simulink model "SWC_CGW_type"  (R2021b)
settings: Solver=FixedStepDiscrete  StartTime=0.0  StopTime=10.0  RelTol=1e-3
(part 2 of 3)

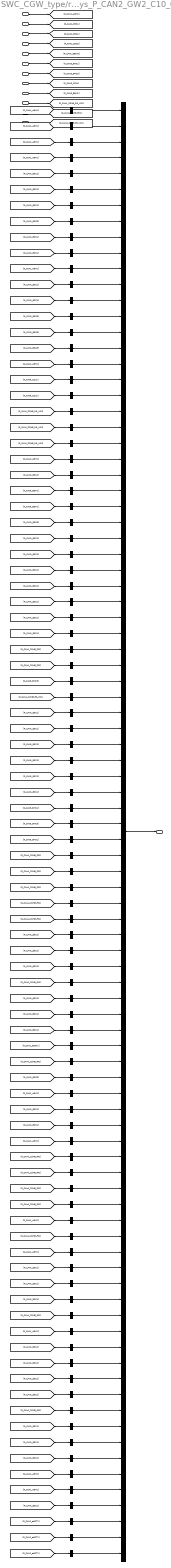
== system SWC_CGW_type/run_SWC_CGW_sys/CGW/Sys_P_CAN2_GW2_C10_0 ==
  R_CAN1_ABM1 : Inport
  R_CAN1_EPS1 : Inport  Port=2
  R_CAN1_ESC1 : Inport  Port=3
  R_CAN1_ESC5 : Inport  Port=4
  R_CAN1_eBST1 : Inport  Port=5
  R_CAN3_BMS1 : Inport  Port=6
  R_CAN3_BMS3 : Inport  Port=7
  R_CAN3_CCU1 : Inport  Port=8
  R_CAN3_EBM1 : Inport  Port=9
  R_CAN4_ZONE_DR_VCU : Inport  Port=10
  R_CAN4_ZONE_FR1 : Inport  Port=11
  R_CAN4_ZONE_FR_VCU : Inport  Port=12
  bus_creator : BusCreator  Inputs=92  OutDataTypeStr=Bus: DT_CAN2_SG_GW2_C10_0  NonVirtualBus=on
  bus_selector : BusSelector  OutputSignals=CAN1_ABM_Passenger_ODS_Sta
  bus_selector1 : BusSelector  OutputSignals=CAN1_ABM_RearPassengerCTR_ODS_Sta
  bus_selector10 : BusSelector  OutputSignals=CAN1_AirBagFailCmd
  bus_selector11 : BusSelector  OutputSignals=CAN1_Amber_WnlmpSta
  bus_selector12 : BusSelector  OutputSignals=CAN1_BTCS_Active
  bus_selector13 : BusSelector  OutputSignals=CAN1_BrkDiscTempSta
  bus_selector14 : BusSelector  OutputSignals=CAN1_BrkSw_Sta
  bus_selector15 : BusSelector  OutputSignals=CAN1_BrkSw_V
  bus_selector16 : BusSelector  OutputSignals=CAN1_CrashOutputSts
  bus_selector17 : BusSelector  OutputSignals=CAN3_DCDCAuxCur
  bus_selector18 : BusSelector  OutputSignals=CAN3_DCDCAuxVolt
  bus_selector19 : BusSelector  OutputSignals=CAN4_DrPMMLVOutPErrLmp
  bus_selector2 : BusSelector  OutputSignals=CAN1_ABM_RearPassengerLH_ODS_Sta
  bus_selector20 : BusSelector  OutputSignals=CAN4_DrPMMSysErrLmp
  bus_selector21 : BusSelector  OutputSignals=CAN4_DrSCPSysErrLmp
  bus_selector22 : BusSelector  OutputSignals=CAN1_DriverSeatBeltCmd
  bus_selector23 : BusSelector  OutputSignals=CAN1_EBD_Failed
  bus_selector24 : BusSelector  OutputSignals=CAN3_EBMErrSta
  bus_selector25 : BusSelector  OutputSignals=CAN3_EBMRLampSta
  bus_selector26 : BusSelector  OutputSignals=CAN1_ESC_ADAS_Sta
  bus_selector27 : BusSelector  OutputSignals=CAN1_ESC_BeepReq
  bus_selector28 : BusSelector  OutputSignals=CAN1_ESC_Failed
  bus_selector29 : BusSelector  OutputSignals=CAN1_ESC_OFF_Status
  bus_selector3 : BusSelector  OutputSignals=CAN1_ABM_RearPassengerRH_ODS_Sta
  bus_selector30 : BusSelector  OutputSignals=CAN1_ESC_Off_lmpSta
  bus_selector31 : BusSelector  OutputSignals=CAN1_ESC_WnlmpSta
  bus_selector32 : BusSelector  OutputSignals=CAN1_ESS_Active
  bus_selector33 : BusSelector  OutputSignals=CAN1_EpasFailed
  bus_selector34 : BusSelector  OutputSignals=CAN4_FLTurn_Light_Warning
  bus_selector35 : BusSelector  OutputSignals=CAN4_FRTurn_Light_Warning
  bus_selector36 : BusSelector  OutputSignals=CAN3_FireDetErr
  bus_selector37 : BusSelector  OutputSignals=CAN4_FrPMMLimpHomeActReq
  bus_selector38 : BusSelector  OutputSignals=CAN1_HBB_Active
  bus_selector39 : BusSelector  OutputSignals=CAN1_HBB_Failed
  bus_selector4 : BusSelector  OutputSignals=CAN1_ABS_Active
  bus_selector40 : BusSelector  OutputSignals=CAN1_HDD_Active
  bus_selector41 : BusSelector  OutputSignals=CAN1_HDD_Failed
  bus_selector42 : BusSelector  OutputSignals=CAN1_HSA_Active
  bus_selector43 : BusSelector  OutputSignals=CAN1_HSA_Failed
  bus_selector44 : BusSelector  OutputSignals=CAN3_HVBattCurr
  bus_selector45 : BusSelector  OutputSignals=CAN3_HVBattErr
  bus_selector46 : BusSelector  OutputSignals=CAN3_HVBattVolt
  bus_selector47 : BusSelector  OutputSignals=CAN4_LADB_Hibeam_Indication
  bus_selector48 : BusSelector  OutputSignals=CAN4_LADB_Operation_Status
  bus_selector49 : BusSelector  OutputSignals=CAN4_LADB_Warning
  bus_selector5 : BusSelector  OutputSignals=CAN1_ABS_Failed
  bus_selector50 : BusSelector  OutputSignals=CAN4_LAHB_Warning
  bus_selector51 : BusSelector  OutputSignals=CAN4_LDRL_Warning
  bus_selector52 : BusSelector  OutputSignals=CAN1_LF_PulseCount
  bus_selector53 : BusSelector  OutputSignals=CAN1_LF_PulseCount_V
  bus_selector54 : BusSelector  OutputSignals=CAN1_LF_WhlRotDir
  bus_selector55 : BusSelector  OutputSignals=CAN4_LLB_Warning
  bus_selector56 : BusSelector  OutputSignals=CAN1_LR_PulseCount
  bus_selector57 : BusSelector  OutputSignals=CAN1_LR_PulseCount_V
  bus_selector58 : BusSelector  OutputSignals=CAN1_LR_WhlRotDir
  bus_selector59 : BusSelector  OutputSignals=CAN1_LowBrakeFluid_Sta
  bus_selector6 : BusSelector  OutputSignals=CAN1_ABS_WnlmpSta
  bus_selector60 : BusSelector  OutputSignals=CAN4_Lposition_Lamp_Warning
  bus_selector61 : BusSelector  OutputSignals=CAN1_Meter_Ind_VehSpeed
  bus_selector62 : BusSelector  OutputSignals=CAN1_PABSwitchCmd
  bus_selector63 : BusSelector  OutputSignals=CAN1_PBA_Active
  bus_selector64 : BusSelector  OutputSignals=CAN1_PBA_Failed
  bus_selector65 : BusSelector  OutputSignals=CAN1_PsngrSeatBeltCmd
  bus_selector66 : BusSelector  OutputSignals=CAN4_RADB_Hibeam_Indication
  bus_selector67 : BusSelector  OutputSignals=CAN4_RADB_Operation_Status
  bus_selector68 : BusSelector  OutputSignals=CAN4_RADB_Warning
  bus_selector69 : BusSelector  OutputSignals=CAN4_RAHB_Warning
  bus_selector7 : BusSelector  OutputSignals=CAN1_AEBAvail
  bus_selector70 : BusSelector  OutputSignals=CAN1_RCenterSeatBeltCmd
  bus_selector71 : BusSelector  OutputSignals=CAN4_RDRL_Warning
  bus_selector72 : BusSelector  OutputSignals=CAN1_RDriverSeatBeltCmd
  bus_selector73 : BusSelector  OutputSignals=CAN1_RF_PulseCount
  bus_selector74 : BusSelector  OutputSignals=CAN1_RF_PulseCount_V
  bus_selector75 : BusSelector  OutputSignals=CAN1_RF_WhlRotDir
  bus_selector76 : BusSelector  OutputSignals=CAN4_RLB_Warning
  bus_selector77 : BusSelector  OutputSignals=CAN1_RPsngrSeatBeltCmd
  bus_selector78 : BusSelector  OutputSignals=CAN1_RR_PulseCount
  bus_selector79 : BusSelector  OutputSignals=CAN1_RR_PulseCount_V
  bus_selector8 : BusSelector  OutputSignals=CAN1_AVH_Active
  bus_selector80 : BusSelector  OutputSignals=CAN1_RR_WhlRotDir
  bus_selector81 : BusSelector  OutputSignals=CAN1_Red_WnlmpSta
  bus_selector82 : BusSelector  OutputSignals=CAN4_Rposition_Lamp_Warning
  bus_selector83 : BusSelector  OutputSignals=CAN1_SAS_Angle
  bus_selector84 : BusSelector  OutputSignals=CAN1_SAS_V
  bus_selector85 : BusSelector  OutputSignals=CAN1_TCS_Failed
  bus_selector86 : BusSelector  OutputSignals=CAN1_TLHPsngrSeatBeltCmd
  bus_selector87 : BusSelector  OutputSignals=CAN1_TRHPsngrSeatBeltCmd
  bus_selector88 : BusSelector  OutputSignals=CAN1_VehSpeed
  bus_selector89 : BusSelector  OutputSignals=CAN1_eBST_AmberWnlmpSta
  bus_selector9 : BusSelector  OutputSignals=CAN1_AVH_Failed
  bus_selector90 : BusSelector  OutputSignals=CAN1_eBST_BeepReq
  bus_selector91 : BusSelector  OutputSignals=CAN1_eBST_RedWnlmpSta
  P_CAN2_GW2_C10_0 : Outport
  wires:
  bus_creator/1 -> P_CAN2_GW2_C10_0/1
  bus_selector/1 -> bus_creator/1  "<CAN1_ABM_Passenger_ODS_Sta>"
  [R_CAN1_ABM1] -> bus_selector/1
  bus_selector1/1 -> bus_creator/2  "<CAN1_ABM_RearPassengerCTR_ODS_Sta>"
  [R_CAN1_ABM1] -> bus_selector1/1
  bus_selector2/1 -> bus_creator/3  "<CAN1_ABM_RearPassengerLH_ODS_Sta>"
  [R_CAN1_ABM1] -> bus_selector2/1
  bus_selector3/1 -> bus_creator/4  "<CAN1_ABM_RearPassengerRH_ODS_Sta>"
  [R_CAN1_ABM1] -> bus_selector3/1
  bus_selector4/1 -> bus_creator/5  "<CAN1_ABS_Active>"
  [R_CAN1_ESC1] -> bus_selector4/1
  bus_selector5/1 -> bus_creator/6  "<CAN1_ABS_Failed>"
  [R_CAN1_ESC1] -> bus_selector5/1
  bus_selector6/1 -> bus_creator/7  "<CAN1_ABS_WnlmpSta>"
  [R_CAN1_ESC1] -> bus_selector6/1
  bus_selector7/1 -> bus_creator/8  "<CAN1_AEBAvail>"
  [R_CAN1_ESC5] -> bus_selector7/1
  bus_selector8/1 -> bus_creator/9  "<CAN1_AVH_Active>"
  [R_CAN1_ESC1] -> bus_selector8/1
  bus_selector9/1 -> bus_creator/10  "<CAN1_AVH_Failed>"
  [R_CAN1_ESC1] -> bus_selector9/1
  bus_selector10/1 -> bus_creator/11  "<CAN1_AirBagFailCmd>"
  [R_CAN1_ABM1] -> bus_selector10/1
  bus_selector11/1 -> bus_creator/12  "<CAN1_Amber_WnlmpSta>"
  [R_CAN1_ESC1] -> bus_selector11/1
  bus_selector12/1 -> bus_creator/13  "<CAN1_BTCS_Active>"
  [R_CAN1_ESC1] -> bus_selector12/1
  bus_selector13/1 -> bus_creator/14  "<CAN1_BrkDiscTempSta>"
  [R_CAN1_ESC5] -> bus_selector13/1
  bus_selector14/1 -> bus_creator/15  "<CAN1_BrkSw_Sta>"
  [R_CAN1_ESC5] -> bus_selector14/1
  bus_selector15/1 -> bus_creator/16  "<CAN1_BrkSw_V>"
  [R_CAN1_ESC5] -> bus_selector15/1
  bus_selector16/1 -> bus_creator/17  "<CAN1_CrashOutputSts>"
  [R_CAN1_ABM1] -> bus_selector16/1
  bus_selector17/1 -> bus_creator/18  "<CAN3_DCDCAuxCur>"
  [R_CAN3_CCU1] -> bus_selector17/1
  bus_selector18/1 -> bus_creator/19  "<CAN3_DCDCAuxVolt>"
  [R_CAN3_CCU1] -> bus_selector18/1
  bus_selector19/1 -> bus_creator/20  "<CAN4_DrPMMLVOutPErrLmp>"
  [R_CAN4_ZONE_DR_VCU] -> bus_selector19/1
  bus_selector20/1 -> bus_creator/21  "<CAN4_DrPMMSysErrLmp>"
  [R_CAN4_ZONE_DR_VCU] -> bus_selector20/1
  bus_selector21/1 -> bus_creator/22  "<CAN4_DrSCPSysErrLmp>"
  [R_CAN4_ZONE_DR_VCU] -> bus_selector21/1
  bus_selector22/1 -> bus_creator/23  "<CAN1_DriverSeatBeltCmd>"
  [R_CAN1_ABM1] -> bus_selector22/1
  bus_selector23/1 -> bus_creator/24  "<CAN1_EBD_Failed>"
  [R_CAN1_ESC1] -> bus_selector23/1
  bus_selector24/1 -> bus_creator/25  "<CAN3_EBMErrSta>"
  [R_CAN3_EBM1] -> bus_selector24/1
  bus_selector25/1 -> bus_creator/26  "<CAN3_EBMRLampSta>"
  [R_CAN3_EBM1] -> bus_selector25/1
  bus_selector26/1 -> bus_creator/27  "<CAN1_ESC_ADAS_Sta>"
  [R_CAN1_ESC5] -> bus_selector26/1
  bus_selector27/1 -> bus_creator/28  "<CAN1_ESC_BeepReq>"
  [R_CAN1_ESC1] -> bus_selector27/1
  bus_selector28/1 -> bus_creator/29  "<CAN1_ESC_Failed>"
  [R_CAN1_ESC1] -> bus_selector28/1
  bus_selector29/1 -> bus_creator/30  "<CAN1_ESC_OFF_Status>"
  [R_CAN1_ESC1] -> bus_selector29/1
  bus_selector30/1 -> bus_creator/31  "<CAN1_ESC_Off_lmpSta>"
  [R_CAN1_ESC1] -> bus_selector30/1
  bus_selector31/1 -> bus_creator/32  "<CAN1_ESC_WnlmpSta>"
  [R_CAN1_ESC1] -> bus_selector31/1
  bus_selector32/1 -> bus_creator/33  "<CAN1_ESS_Active>"
  [R_CAN1_ESC1] -> bus_selector32/1
  bus_selector33/1 -> bus_creator/34  "<CAN1_EpasFailed>"
  [R_CAN1_EPS1] -> bus_selector33/1
  bus_selector34/1 -> bus_creator/35  "<CAN4_FLTurn_Light_Warning>"
  [R_CAN4_ZONE_FR1] -> bus_selector34/1
  bus_selector35/1 -> bus_creator/36  "<CAN4_FRTurn_Light_Warning>"
  [R_CAN4_ZONE_FR1] -> bus_selector35/1
  bus_selector36/1 -> bus_creator/37  "<CAN3_FireDetErr>"
  [R_CAN3_BMS3] -> bus_selector36/1
  bus_selector37/1 -> bus_creator/38  "<CAN4_FrPMMLimpHomeActReq>"
  [R_CAN4_ZONE_FR_VCU] -> bus_selector37/1
  bus_selector38/1 -> bus_creator/39  "<CAN1_HBB_Active>"
  [R_CAN1_ESC1] -> bus_selector38/1
  bus_selector39/1 -> bus_creator/40  "<CAN1_HBB_Failed>"
  [R_CAN1_ESC1] -> bus_selector39/1
  bus_selector40/1 -> bus_creator/41  "<CAN1_HDD_Active>"
  [R_CAN1_ESC1] -> bus_selector40/1
  bus_selector41/1 -> bus_creator/42  "<CAN1_HDD_Failed>"
  [R_CAN1_ESC1] -> bus_selector41/1
  bus_selector42/1 -> bus_creator/43  "<CAN1_HSA_Active>"
  [R_CAN1_ESC1] -> bus_selector42/1
  bus_selector43/1 -> bus_creator/44  "<CAN1_HSA_Failed>"
  [R_CAN1_ESC1] -> bus_selector43/1
  bus_selector44/1 -> bus_creator/45  "<CAN3_HVBattCurr>"
  [R_CAN3_BMS1] -> bus_selector44/1
  bus_selector45/1 -> bus_creator/46  "<CAN3_HVBattErr>"
  [R_CAN3_BMS3] -> bus_selector45/1
  bus_selector46/1 -> bus_creator/47  "<CAN3_HVBattVolt>"
  [R_CAN3_BMS1] -> bus_selector46/1
  bus_selector47/1 -> bus_creator/48  "<CAN4_LADB_Hibeam_Indication>"
  [R_CAN4_ZONE_FR1] -> bus_selector47/1
  bus_selector48/1 -> bus_creator/49  "<CAN4_LADB_Operation_Status>"
  [R_CAN4_ZONE_FR1] -> bus_selector48/1
  bus_selector49/1 -> bus_creator/50  "<CAN4_LADB_Warning>"
  [R_CAN4_ZONE_FR1] -> bus_selector49/1
  bus_selector50/1 -> bus_creator/51  "<CAN4_LAHB_Warning>"
  [R_CAN4_ZONE_FR1] -> bus_selector50/1
  bus_selector51/1 -> bus_creator/52  "<CAN4_LDRL_Warning>"
  [R_CAN4_ZONE_FR1] -> bus_selector51/1
  bus_selector52/1 -> bus_creator/53  "<CAN1_LF_PulseCount>"
  [R_CAN1_ESC1] -> bus_selector52/1
  bus_selector53/1 -> bus_creator/54  "<CAN1_LF_PulseCount_V>"
  [R_CAN1_ESC1] -> bus_selector53/1
  bus_selector54/1 -> bus_creator/55  "<CAN1_LF_WhlRotDir>"
  [R_CAN1_ESC1] -> bus_selector54/1
  bus_selector55/1 -> bus_creator/56  "<CAN4_LLB_Warning>"
  [R_CAN4_ZONE_FR1] -> bus_selector55/1
  bus_selector56/1 -> bus_creator/57  "<CAN1_LR_PulseCount>"
  [R_CAN1_ESC1] -> bus_selector56/1
  bus_selector57/1 -> bus_creator/58  "<CAN1_LR_PulseCount_V>"
  [R_CAN1_ESC1] -> bus_selector57/1
  bus_selector58/1 -> bus_creator/59  "<CAN1_LR_WhlRotDir>"
  [R_CAN1_ESC1] -> bus_selector58/1
  bus_selector59/1 -> bus_creator/60  "<CAN1_LowBrakeFluid_Sta>"
  [R_CAN1_eBST1] -> bus_selector59/1
  bus_selector60/1 -> bus_creator/61  "<CAN4_Lposition_Lamp_Warning>"
  [R_CAN4_ZONE_FR1] -> bus_selector60/1
  bus_selector61/1 -> bus_creator/62  "<CAN1_Meter_Ind_VehSpeed>"
  [R_CAN1_ESC5] -> bus_selector61/1
  bus_selector62/1 -> bus_creator/63  "<CAN1_PABSwitchCmd>"
  [R_CAN1_ABM1] -> bus_selector62/1
  bus_selector63/1 -> bus_creator/64  "<CAN1_PBA_Active>"
  [R_CAN1_ESC1] -> bus_selector63/1
  bus_selector64/1 -> bus_creator/65  "<CAN1_PBA_Failed>"
  [R_CAN1_ESC1] -> bus_selector64/1
  bus_selector65/1 -> bus_creator/66  "<CAN1_PsngrSeatBeltCmd>"
  [R_CAN1_ABM1] -> bus_selector65/1
  bus_selector66/1 -> bus_creator/67  "<CAN4_RADB_Hibeam_Indication>"
  [R_CAN4_ZONE_FR1] -> bus_selector66/1
  bus_selector67/1 -> bus_creator/68  "<CAN4_RADB_Operation_Status>"
  [R_CAN4_ZONE_FR1] -> bus_selector67/1
  bus_selector68/1 -> bus_creator/69  "<CAN4_RADB_Warning>"
  [R_CAN4_ZONE_FR1] -> bus_selector68/1
  bus_selector69/1 -> bus_creator/70  "<CAN4_RAHB_Warning>"
  [R_CAN4_ZONE_FR1] -> bus_selector69/1
  bus_selector70/1 -> bus_creator/71  "<CAN1_RCenterSeatBeltCmd>"
  [R_CAN1_ABM1] -> bus_selector70/1
  bus_selector71/1 -> bus_creator/72  "<CAN4_RDRL_Warning>"
  [R_CAN4_ZONE_FR1] -> bus_selector71/1
  bus_selector72/1 -> bus_creator/73  "<CAN1_RDriverSeatBeltCmd>"
  [R_CAN1_ABM1] -> bus_selector72/1
  bus_selector73/1 -> bus_creator/74  "<CAN1_RF_PulseCount>"
  [R_CAN1_ESC1] -> bus_selector73/1
  bus_selector74/1 -> bus_creator/75  "<CAN1_RF_PulseCount_V>"
  [R_CAN1_ESC1] -> bus_selector74/1
  bus_selector75/1 -> bus_creator/76  "<CAN1_RF_WhlRotDir>"
  [R_CAN1_ESC1] -> bus_selector75/1
  bus_selector76/1 -> bus_creator/77  "<CAN4_RLB_Warning>"
  [R_CAN4_ZONE_FR1] -> bus_selector76/1
  bus_selector77/1 -> bus_creator/78  "<CAN1_RPsngrSeatBeltCmd>"
  [R_CAN1_ABM1] -> bus_selector77/1
  bus_selector78/1 -> bus_creator/79  "<CAN1_RR_PulseCount>"
  [R_CAN1_ESC1] -> bus_selector78/1
  bus_selector79/1 -> bus_creator/80  "<CAN1_RR_PulseCount_V>"
  [R_CAN1_ESC1] -> bus_selector79/1
  bus_selector80/1 -> bus_creator/81  "<CAN1_RR_WhlRotDir>"
  [R_CAN1_ESC1] -> bus_selector80/1
  bus_selector81/1 -> bus_creator/82  "<CAN1_Red_WnlmpSta>"
  [R_CAN1_ESC1] -> bus_selector81/1
  bus_selector82/1 -> bus_creator/83  "<CAN4_Rposition_Lamp_Warning>"
  [R_CAN4_ZONE_FR1] -> bus_selector82/1
  bus_selector83/1 -> bus_creator/84  "<CAN1_SAS_Angle>"
  [R_CAN1_EPS1] -> bus_selector83/1
  bus_selector84/1 -> bus_creator/85  "<CAN1_SAS_V>"
  [R_CAN1_EPS1] -> bus_selector84/1
  bus_selector85/1 -> bus_creator/86  "<CAN1_TCS_Failed>"
  [R_CAN1_ESC1] -> bus_selector85/1
  bus_selector86/1 -> bus_creator/87  "<CAN1_TLHPsngrSeatBeltCmd>"
  [R_CAN1_ABM1] -> bus_selector86/1
  bus_selector87/1 -> bus_creator/88  "<CAN1_TRHPsngrSeatBeltCmd>"
  [R_CAN1_ABM1] -> bus_selector87/1
  bus_selector88/1 -> bus_creator/89  "<CAN1_VehSpeed>"
  [R_CAN1_ESC1] -> bus_selector88/1
  bus_selector89/1 -> bus_creator/90  "<CAN1_eBST_AmberWnlmpSta>"
  [R_CAN1_eBST1] -> bus_selector89/1
  bus_selector90/1 -> bus_creator/91  "<CAN1_eBST_BeepReq>"
  [R_CAN1_eBST1] -> bus_selector90/1
  bus_selector91/1 -> bus_creator/92  "<CAN1_eBST_RedWnlmpSta>"
  [R_CAN1_eBST1] -> bus_selector91/1
  R_CAN1_ABM1/1 -> [R_CAN1_ABM1]
  R_CAN1_EPS1/1 -> [R_CAN1_EPS1]
  R_CAN1_ESC1/1 -> [R_CAN1_ESC1]
  R_CAN1_ESC5/1 -> [R_CAN1_ESC5]
  R_CAN1_eBST1/1 -> [R_CAN1_eBST1]
  R_CAN3_BMS1/1 -> [R_CAN3_BMS1]
  R_CAN3_BMS3/1 -> [R_CAN3_BMS3]
  R_CAN3_CCU1/1 -> [R_CAN3_CCU1]
  R_CAN3_EBM1/1 -> [R_CAN3_EBM1]
  R_CAN4_ZONE_DR_VCU/1 -> [R_CAN4_ZONE_DR_VCU]
  R_CAN4_ZONE_FR1/1 -> [R_CAN4_ZONE_FR1]
  R_CAN4_ZONE_FR_VCU/1 -> [R_CAN4_ZONE_FR_VCU]

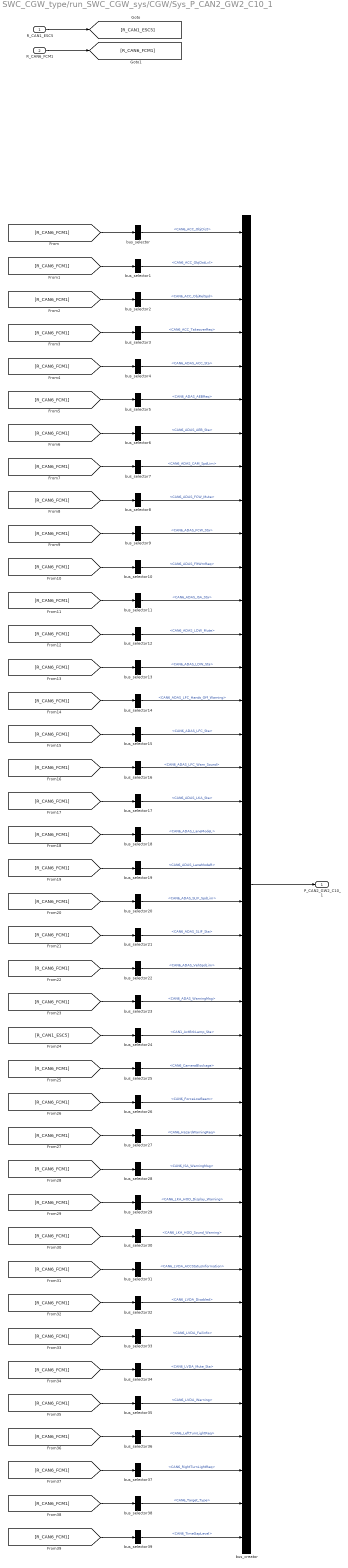
== system SWC_CGW_type/run_SWC_CGW_sys/CGW/Sys_P_CAN2_GW2_C10_1 ==
  R_CAN1_ESC5 : Inport
  R_CAN6_FCM1 : Inport  Port=2
  bus_creator : BusCreator  Inputs=40  OutDataTypeStr=Bus: DT_CAN2_SG_GW2_C10_1  NonVirtualBus=on
  bus_selector : BusSelector  OutputSignals=CAN6_ACC_ObjDist
  bus_selector1 : BusSelector  OutputSignals=CAN6_ACC_ObjDstLvl
  bus_selector10 : BusSelector  OutputSignals=CAN6_ADAS_FltWrnReq
  bus_selector11 : BusSelector  OutputSignals=CAN6_ADAS_ISA_Sta
  bus_selector12 : BusSelector  OutputSignals=CAN6_ADAS_LDW_Mute
  bus_selector13 : BusSelector  OutputSignals=CAN6_ADAS_LDW_Sta
  bus_selector14 : BusSelector  OutputSignals=CAN6_ADAS_LFC_Hands_Off_Warning
  bus_selector15 : BusSelector  OutputSignals=CAN6_ADAS_LFC_Sta
  bus_selector16 : BusSelector  OutputSignals=CAN6_ADAS_LFC_Warn_Sound
  bus_selector17 : BusSelector  OutputSignals=CAN6_ADAS_LKA_Sta
  bus_selector18 : BusSelector  OutputSignals=CAN6_ADAS_LaneModeL
  bus_selector19 : BusSelector  OutputSignals=CAN6_ADAS_LaneModeR
  bus_selector2 : BusSelector  OutputSignals=CAN6_ACC_ObjRelSpd
  bus_selector20 : BusSelector  OutputSignals=CAN6_ADAS_SLIF_SpdLim
  bus_selector21 : BusSelector  OutputSignals=CAN6_ADAS_SLIF_Sta
  bus_selector22 : BusSelector  OutputSignals=CAN6_ADAS_VehSpdLim
  bus_selector23 : BusSelector  OutputSignals=CAN6_ADAS_WarningMsg
  bus_selector24 : BusSelector  OutputSignals=CAN1_ActBrkLamp_Sta
  bus_selector25 : BusSelector  OutputSignals=CAN6_CameraBlockage
  bus_selector26 : BusSelector  OutputSignals=CAN6_ForceLowBeam
  bus_selector27 : BusSelector  OutputSignals=CAN6_HazardWarningReq
  bus_selector28 : BusSelector  OutputSignals=CAN6_ISA_WarningMsg
  bus_selector29 : BusSelector  OutputSignals=CAN6_LKA_HOD_Display_Warning
  bus_selector3 : BusSelector  OutputSignals=CAN6_ACC_TakeoverReq
  bus_selector30 : BusSelector  OutputSignals=CAN6_LKA_HOD_Sound_Warning
  bus_selector31 : BusSelector  OutputSignals=CAN6_LVDA_ACCStatusInformation
  bus_selector32 : BusSelector  OutputSignals=CAN6_LVDA_Disabled
  bus_selector33 : BusSelector  OutputSignals=CAN6_LVDA_Failinfo
  bus_selector34 : BusSelector  OutputSignals=CAN6_LVDA_Mute_Sta
  bus_selector35 : BusSelector  OutputSignals=CAN6_LVDA_Warning
  bus_selector36 : BusSelector  OutputSignals=CAN6_LeftTurnLightReq
  bus_selector37 : BusSelector  OutputSignals=CAN6_RightTurnLightReq
  bus_selector38 : BusSelector  OutputSignals=CAN6_Target_Type
  bus_selector39 : BusSelector  OutputSignals=CAN6_TimeGapLevel
  bus_selector4 : BusSelector  OutputSignals=CAN6_ADAS_ACC_Sta
  bus_selector5 : BusSelector  OutputSignals=CAN6_ADAS_AEBReq
  bus_selector6 : BusSelector  OutputSignals=CAN6_ADAS_AEB_Sta
  bus_selector7 : BusSelector  OutputSignals=CAN6_ADAS_CAM_SpdLim
  bus_selector8 : BusSelector  OutputSignals=CAN6_ADAS_FCW_Mute
  bus_selector9 : BusSelector  OutputSignals=CAN6_ADAS_FCW_Sta
  P_CAN2_GW2_C10_1 : Outport
  wires:
  bus_creator/1 -> P_CAN2_GW2_C10_1/1
  bus_selector/1 -> bus_creator/1  "<CAN6_ACC_ObjDist>"
  [R_CAN6_FCM1] -> bus_selector/1
  bus_selector1/1 -> bus_creator/2  "<CAN6_ACC_ObjDstLvl>"
  [R_CAN6_FCM1] -> bus_selector1/1
  bus_selector2/1 -> bus_creator/3  "<CAN6_ACC_ObjRelSpd>"
  [R_CAN6_FCM1] -> bus_selector2/1
  bus_selector3/1 -> bus_creator/4  "<CAN6_ACC_TakeoverReq>"
  [R_CAN6_FCM1] -> bus_selector3/1
  bus_selector4/1 -> bus_creator/5  "<CAN6_ADAS_ACC_Sta>"
  [R_CAN6_FCM1] -> bus_selector4/1
  bus_selector5/1 -> bus_creator/6  "<CAN6_ADAS_AEBReq>"
  [R_CAN6_FCM1] -> bus_selector5/1
  bus_selector6/1 -> bus_creator/7  "<CAN6_ADAS_AEB_Sta>"
  [R_CAN6_FCM1] -> bus_selector6/1
  bus_selector7/1 -> bus_creator/8  "<CAN6_ADAS_CAM_SpdLim>"
  [R_CAN6_FCM1] -> bus_selector7/1
  bus_selector8/1 -> bus_creator/9  "<CAN6_ADAS_FCW_Mute>"
  [R_CAN6_FCM1] -> bus_selector8/1
  bus_selector9/1 -> bus_creator/10  "<CAN6_ADAS_FCW_Sta>"
  [R_CAN6_FCM1] -> bus_selector9/1
  bus_selector10/1 -> bus_creator/11  "<CAN6_ADAS_FltWrnReq>"
  [R_CAN6_FCM1] -> bus_selector10/1
  bus_selector11/1 -> bus_creator/12  "<CAN6_ADAS_ISA_Sta>"
  [R_CAN6_FCM1] -> bus_selector11/1
  bus_selector12/1 -> bus_creator/13  "<CAN6_ADAS_LDW_Mute>"
  [R_CAN6_FCM1] -> bus_selector12/1
  bus_selector13/1 -> bus_creator/14  "<CAN6_ADAS_LDW_Sta>"
  [R_CAN6_FCM1] -> bus_selector13/1
  bus_selector14/1 -> bus_creator/15  "<CAN6_ADAS_LFC_Hands_Off_Warning>"
  [R_CAN6_FCM1] -> bus_selector14/1
  bus_selector15/1 -> bus_creator/16  "<CAN6_ADAS_LFC_Sta>"
  [R_CAN6_FCM1] -> bus_selector15/1
  bus_selector16/1 -> bus_creator/17  "<CAN6_ADAS_LFC_Warn_Sound>"
  [R_CAN6_FCM1] -> bus_selector16/1
  bus_selector17/1 -> bus_creator/18  "<CAN6_ADAS_LKA_Sta>"
  [R_CAN6_FCM1] -> bus_selector17/1
  bus_selector18/1 -> bus_creator/19  "<CAN6_ADAS_LaneModeL>"
  [R_CAN6_FCM1] -> bus_selector18/1
  bus_selector19/1 -> bus_creator/20  "<CAN6_ADAS_LaneModeR>"
  [R_CAN6_FCM1] -> bus_selector19/1
  bus_selector20/1 -> bus_creator/21  "<CAN6_ADAS_SLIF_SpdLim>"
  [R_CAN6_FCM1] -> bus_selector20/1
  bus_selector21/1 -> bus_creator/22  "<CAN6_ADAS_SLIF_Sta>"
  [R_CAN6_FCM1] -> bus_selector21/1
  bus_selector22/1 -> bus_creator/23  "<CAN6_ADAS_VehSpdLim>"
  [R_CAN6_FCM1] -> bus_selector22/1
  bus_selector23/1 -> bus_creator/24  "<CAN6_ADAS_WarningMsg>"
  [R_CAN6_FCM1] -> bus_selector23/1
  bus_selector24/1 -> bus_creator/25  "<CAN1_ActBrkLamp_Sta>"
  [R_CAN1_ESC5] -> bus_selector24/1
  bus_selector25/1 -> bus_creator/26  "<CAN6_CameraBlockage>"
  [R_CAN6_FCM1] -> bus_selector25/1
  bus_selector26/1 -> bus_creator/27  "<CAN6_ForceLowBeam>"
  [R_CAN6_FCM1] -> bus_selector26/1
  bus_selector27/1 -> bus_creator/28  "<CAN6_HazardWarningReq>"
  [R_CAN6_FCM1] -> bus_selector27/1
  bus_selector28/1 -> bus_creator/29  "<CAN6_ISA_WarningMsg>"
  [R_CAN6_FCM1] -> bus_selector28/1
  bus_selector29/1 -> bus_creator/30  "<CAN6_LKA_HOD_Display_Warning>"
  [R_CAN6_FCM1] -> bus_selector29/1
  bus_selector30/1 -> bus_creator/31  "<CAN6_LKA_HOD_Sound_Warning>"
  [R_CAN6_FCM1] -> bus_selector30/1
  bus_selector31/1 -> bus_creator/32  "<CAN6_LVDA_ACCStatusInformation>"
  [R_CAN6_FCM1] -> bus_selector31/1
  bus_selector32/1 -> bus_creator/33  "<CAN6_LVDA_Disabled>"
  [R_CAN6_FCM1] -> bus_selector32/1
  bus_selector33/1 -> bus_creator/34  "<CAN6_LVDA_Failinfo>"
  [R_CAN6_FCM1] -> bus_selector33/1
  bus_selector34/1 -> bus_creator/35  "<CAN6_LVDA_Mute_Sta>"
  [R_CAN6_FCM1] -> bus_selector34/1
  bus_selector35/1 -> bus_creator/36  "<CAN6_LVDA_Warning>"
  [R_CAN6_FCM1] -> bus_selector35/1
  bus_selector36/1 -> bus_creator/37  "<CAN6_LeftTurnLightReq>"
  [R_CAN6_FCM1] -> bus_selector36/1
  bus_selector37/1 -> bus_creator/38  "<CAN6_RightTurnLightReq>"
  [R_CAN6_FCM1] -> bus_selector37/1
  bus_selector38/1 -> bus_creator/39  "<CAN6_Target_Type>"
  [R_CAN6_FCM1] -> bus_selector38/1
  bus_selector39/1 -> bus_creator/40  "<CAN6_TimeGapLevel>"
  [R_CAN6_FCM1] -> bus_selector39/1
  R_CAN1_ESC5/1 -> [R_CAN1_ESC5]
  R_CAN6_FCM1/1 -> [R_CAN6_FCM1]

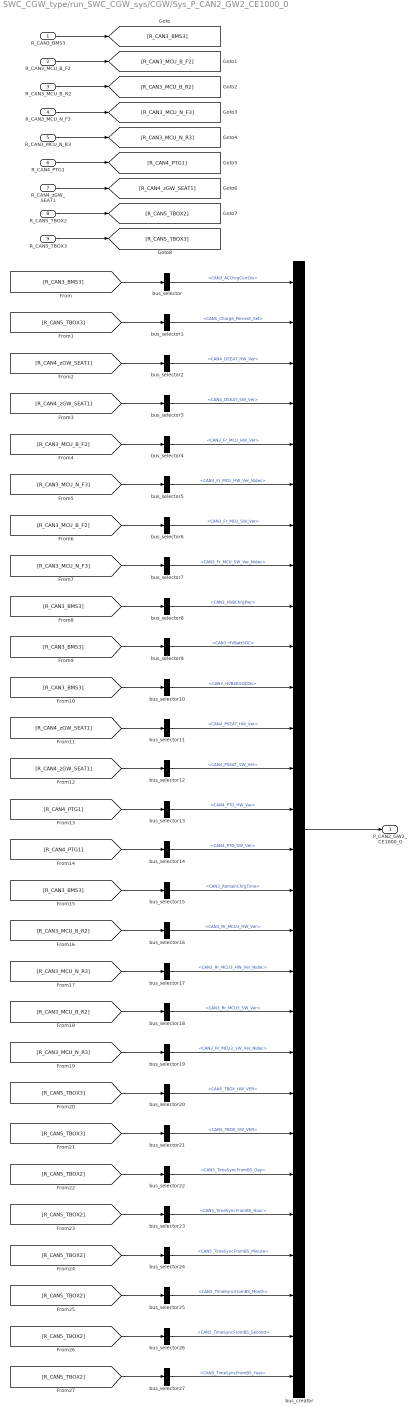
== system SWC_CGW_type/run_SWC_CGW_sys/CGW/Sys_P_CAN2_GW2_CE1000_0 ==
  R_CAN3_BMS3 : Inport
  R_CAN3_MCU_B_F2 : Inport  Port=2
  R_CAN3_MCU_B_R2 : Inport  Port=3
  R_CAN3_MCU_N_F3 : Inport  Port=4
  R_CAN3_MCU_N_R3 : Inport  Port=5
  R_CAN4_PTG1 : Inport  Port=6
  R_CAN4_zGW_SEAT1 : Inport  Port=7
  R_CAN5_TBOX2 : Inport  Port=8
  R_CAN5_TBOX3 : Inport  Port=9
  bus_creator : BusCreator  Inputs=28  OutDataTypeStr=Bus: DT_CAN2_SG_GW2_CE1000_0  NonVirtualBus=on
  bus_selector : BusSelector  OutputSignals=CAN3_ACChrgCurrDis
  bus_selector1 : BusSelector  OutputSignals=CAN5_Charge_Percent_Set
  bus_selector10 : BusSelector  OutputSignals=CAN3_HVBattSOCDis
  bus_selector11 : BusSelector  OutputSignals=CAN4_PSEAT_HW_Ver
  bus_selector12 : BusSelector  OutputSignals=CAN4_PSEAT_SW_Ver
  bus_selector13 : BusSelector  OutputSignals=CAN4_PTG_HW_Ver
  bus_selector14 : BusSelector  OutputSignals=CAN4_PTG_SW_Ver
  bus_selector15 : BusSelector  OutputSignals=CAN3_RemainChrgTime
  bus_selector16 : BusSelector  OutputSignals=CAN3_Rr_MCU3_HW_Ver
  bus_selector17 : BusSelector  OutputSignals=CAN3_Rr_MCU3_HW_Ver_Nidec
  bus_selector18 : BusSelector  OutputSignals=CAN3_Rr_MCU3_SW_Ver
  bus_selector19 : BusSelector  OutputSignals=CAN3_Rr_MCU3_SW_Ver_Nidec
  bus_selector2 : BusSelector  OutputSignals=CAN4_DSEAT_HW_Ver
  bus_selector20 : BusSelector  OutputSignals=CAN5_TBOX_HW_VER
  bus_selector21 : BusSelector  OutputSignals=CAN5_TBOX_SW_VER
  bus_selector22 : BusSelector  OutputSignals=CAN5_TimeSyncFromBS_Day
  bus_selector23 : BusSelector  OutputSignals=CAN5_TimeSyncFromBS_Hour
  bus_selector24 : BusSelector  OutputSignals=CAN5_TimeSyncFromBS_Minute
  bus_selector25 : BusSelector  OutputSignals=CAN5_TimeSyncFromBS_Month
  bus_selector26 : BusSelector  OutputSignals=CAN5_TimeSyncFromBS_Second
  bus_selector27 : BusSelector  OutputSignals=CAN5_TimeSyncFromBS_Year
  bus_selector3 : BusSelector  OutputSignals=CAN4_DSEAT_SW_Ver
  bus_selector4 : BusSelector  OutputSignals=CAN3_Fr_MCU_HW_Ver
  bus_selector5 : BusSelector  OutputSignals=CAN3_Fr_MCU_HW_Ver_Nidec
  bus_selector6 : BusSelector  OutputSignals=CAN3_Fr_MCU_SW_Ver
  bus_selector7 : BusSelector  OutputSignals=CAN3_Fr_MCU_SW_Ver_Nidec
  bus_selector8 : BusSelector  OutputSignals=CAN3_HVBChrgPwr
  bus_selector9 : BusSelector  OutputSignals=CAN3_HVBattSOC
  P_CAN2_GW2_CE1000_0 : Outport
  wires:
  bus_creator/1 -> P_CAN2_GW2_CE1000_0/1
  bus_selector/1 -> bus_creator/1  "<CAN3_ACChrgCurrDis>"
  [R_CAN3_BMS3] -> bus_selector/1
  bus_selector1/1 -> bus_creator/2  "<CAN5_Charge_Percent_Set>"
  [R_CAN5_TBOX3] -> bus_selector1/1
  bus_selector2/1 -> bus_creator/3  "<CAN4_DSEAT_HW_Ver>"
  [R_CAN4_zGW_SEAT1] -> bus_selector2/1
  bus_selector3/1 -> bus_creator/4  "<CAN4_DSEAT_SW_Ver>"
  [R_CAN4_zGW_SEAT1] -> bus_selector3/1
  bus_selector4/1 -> bus_creator/5  "<CAN3_Fr_MCU_HW_Ver>"
  [R_CAN3_MCU_B_F2] -> bus_selector4/1
  bus_selector5/1 -> bus_creator/6  "<CAN3_Fr_MCU_HW_Ver_Nidec>"
  [R_CAN3_MCU_N_F3] -> bus_selector5/1
  bus_selector6/1 -> bus_creator/7  "<CAN3_Fr_MCU_SW_Ver>"
  [R_CAN3_MCU_B_F2] -> bus_selector6/1
  bus_selector7/1 -> bus_creator/8  "<CAN3_Fr_MCU_SW_Ver_Nidec>"
  [R_CAN3_MCU_N_F3] -> bus_selector7/1
  bus_selector8/1 -> bus_creator/9  "<CAN3_HVBChrgPwr>"
  [R_CAN3_BMS3] -> bus_selector8/1
  bus_selector9/1 -> bus_creator/10  "<CAN3_HVBattSOC>"
  [R_CAN3_BMS3] -> bus_selector9/1
  bus_selector10/1 -> bus_creator/11  "<CAN3_HVBattSOCDis>"
  [R_CAN3_BMS3] -> bus_selector10/1
  bus_selector11/1 -> bus_creator/12  "<CAN4_PSEAT_HW_Ver>"
  [R_CAN4_zGW_SEAT1] -> bus_selector11/1
  bus_selector12/1 -> bus_creator/13  "<CAN4_PSEAT_SW_Ver>"
  [R_CAN4_zGW_SEAT1] -> bus_selector12/1
  bus_selector13/1 -> bus_creator/14  "<CAN4_PTG_HW_Ver>"
  [R_CAN4_PTG1] -> bus_selector13/1
  bus_selector14/1 -> bus_creator/15  "<CAN4_PTG_SW_Ver>"
  [R_CAN4_PTG1] -> bus_selector14/1
  bus_selector15/1 -> bus_creator/16  "<CAN3_RemainChrgTime>"
  [R_CAN3_BMS3] -> bus_selector15/1
  bus_selector16/1 -> bus_creator/17  "<CAN3_Rr_MCU3_HW_Ver>"
  [R_CAN3_MCU_B_R2] -> bus_selector16/1
  bus_selector17/1 -> bus_creator/18  "<CAN3_Rr_MCU3_HW_Ver_Nidec>"
  [R_CAN3_MCU_N_R3] -> bus_selector17/1
  bus_selector18/1 -> bus_creator/19  "<CAN3_Rr_MCU3_SW_Ver>"
  [R_CAN3_MCU_B_R2] -> bus_selector18/1
  bus_selector19/1 -> bus_creator/20  "<CAN3_Rr_MCU3_SW_Ver_Nidec>"
  [R_CAN3_MCU_N_R3] -> bus_selector19/1
  bus_selector20/1 -> bus_creator/21  "<CAN5_TBOX_HW_VER>"
  [R_CAN5_TBOX3] -> bus_selector20/1
  bus_selector21/1 -> bus_creator/22  "<CAN5_TBOX_SW_VER>"
  [R_CAN5_TBOX3] -> bus_selector21/1
  bus_selector22/1 -> bus_creator/23  "<CAN5_TimeSyncFromBS_Day>"
  [R_CAN5_TBOX2] -> bus_selector22/1
  bus_selector23/1 -> bus_creator/24  "<CAN5_TimeSyncFromBS_Hour>"
  [R_CAN5_TBOX2] -> bus_selector23/1
  bus_selector24/1 -> bus_creator/25  "<CAN5_TimeSyncFromBS_Minute>"
  [R_CAN5_TBOX2] -> bus_selector24/1
  bus_selector25/1 -> bus_creator/26  "<CAN5_TimeSyncFromBS_Month>"
  [R_CAN5_TBOX2] -> bus_selector25/1
  bus_selector26/1 -> bus_creator/27  "<CAN5_TimeSyncFromBS_Second>"
  [R_CAN5_TBOX2] -> bus_selector26/1
  bus_selector27/1 -> bus_creator/28  "<CAN5_TimeSyncFromBS_Year>"
  [R_CAN5_TBOX2] -> bus_selector27/1
  R_CAN3_BMS3/1 -> [R_CAN3_BMS3]
  R_CAN3_MCU_B_F2/1 -> [R_CAN3_MCU_B_F2]
  R_CAN3_MCU_B_R2/1 -> [R_CAN3_MCU_B_R2]
  R_CAN3_MCU_N_F3/1 -> [R_CAN3_MCU_N_F3]
  R_CAN3_MCU_N_R3/1 -> [R_CAN3_MCU_N_R3]
  R_CAN4_PTG1/1 -> [R_CAN4_PTG1]
  R_CAN4_zGW_SEAT1/1 -> [R_CAN4_zGW_SEAT1]
  R_CAN5_TBOX2/1 -> [R_CAN5_TBOX2]
  R_CAN5_TBOX3/1 -> [R_CAN5_TBOX3]

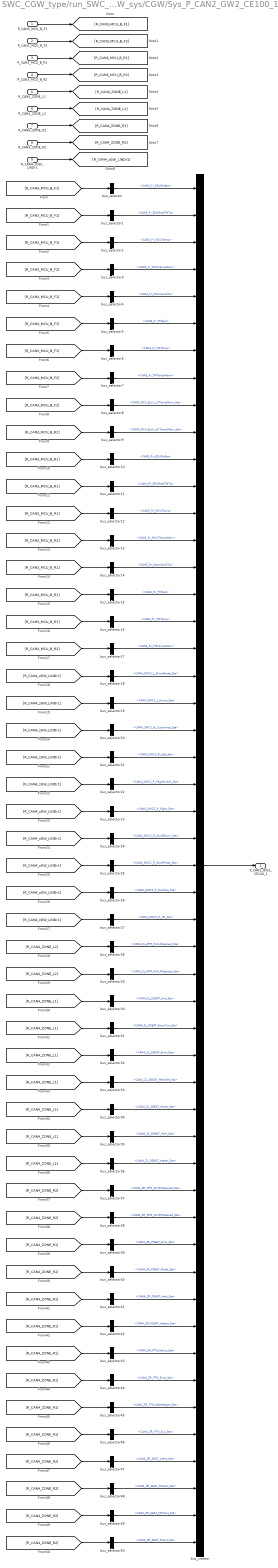
== system SWC_CGW_type/run_SWC_CGW_sys/CGW/Sys_P_CAN2_GW2_CE100_1 ==
  R_CAN3_MCU_B_F1 : Inport
  R_CAN3_MCU_B_F2 : Inport  Port=2
  R_CAN3_MCU_B_R1 : Inport  Port=3
  R_CAN3_MCU_B_R2 : Inport  Port=4
  R_CAN4_ZONE_L1 : Inport  Port=5
  R_CAN4_ZONE_L2 : Inport  Port=6
  R_CAN4_ZONE_R1 : Inport  Port=7
  R_CAN4_ZONE_R2 : Inport  Port=8
  R_CAN4_zGW_LINDr1 : Inport  Port=9
  bus_creator : BusCreator  Inputs=51  OutDataTypeStr=Bus: DT_CAN2_SG_GW2_CE100_1  NonVirtualBus=on
  bus_selector : BusSelector  OutputSignals=CAN3_Fr_EDUDrtSta
  bus_selector1 : BusSelector  OutputSignals=CAN3_Fr_EDURealTMTq
  bus_selector10 : BusSelector  OutputSignals=CAN3_Rr_EDUDrtSta
  bus_selector11 : BusSelector  OutputSignals=CAN3_Rr_EDURealTMTq
  bus_selector12 : BusSelector  OutputSignals=CAN3_Rr_MCUTemp
  bus_selector13 : BusSelector  OutputSignals=CAN3_Rr_MCUTempWarn
  bus_selector14 : BusSelector  OutputSignals=CAN3_Rr_MotorAvailTq
  bus_selector15 : BusSelector  OutputSignals=CAN3_Rr_TMSpd
  bus_selector16 : BusSelector  OutputSignals=CAN3_Rr_TMTemp
  bus_selector17 : BusSelector  OutputSignals=CAN3_Rr_TMTempWarn
  bus_selector18 : BusSelector  OutputSignals=CAN4_SWC2_L_DriveMode_Sta
  bus_selector19 : BusSelector  OutputSignals=CAN4_SWC2_L_Home_Sta
  bus_selector2 : BusSelector  OutputSignals=CAN3_Fr_MCUTemp
  bus_selector20 : BusSelector  OutputSignals=CAN4_SWC2_R_Customize_Sta
  bus_selector21 : BusSelector  OutputSignals=CAN4_SWC2_R_Left_Sta
  bus_selector22 : BusSelector  OutputSignals=CAN4_SWC2_R_PageSwitch_Sta
  bus_selector23 : BusSelector  OutputSignals=CAN4_SWC2_R_Right_Sta
  bus_selector24 : BusSelector  OutputSignals=CAN4_SWC2_R_ScrollDown_Sta
  bus_selector25 : BusSelector  OutputSignals=CAN4_SWC2_R_ScrollPress_Sta
  bus_selector26 : BusSelector  OutputSignals=CAN4_SWC2_R_ScrollUp_Sta
  bus_selector27 : BusSelector  OutputSignals=CAN4_SWC2_R_VR_Sta
  bus_selector28 : BusSelector  OutputSignals=CAN4_ZL_APM_WinLFOpened_Sta
  bus_selector29 : BusSelector  OutputSignals=CAN4_ZL_APM_WinLROpened_Sta
  bus_selector3 : BusSelector  OutputSignals=CAN3_Fr_MCUTempWarn
  bus_selector30 : BusSelector  OutputSignals=CAN4_ZL_DSEAT_Anti_Sta
  bus_selector31 : BusSelector  OutputSignals=CAN4_ZL_DSEAT_EntryFun_Sta
  bus_selector32 : BusSelector  OutputSignals=CAN4_ZL_DSEAT_Error_Sta
  bus_selector33 : BusSelector  OutputSignals=CAN4_ZL_DSEAT_MemSet_Sta
  bus_selector34 : BusSelector  OutputSignals=CAN4_ZL_DSEAT_Mode_Sta
  bus_selector35 : BusSelector  OutputSignals=CAN4_ZL_DSEAT_Vent_Sta
  bus_selector36 : BusSelector  OutputSignals=CAN4_ZL_DSEAT_heater_Sta
  bus_selector37 : BusSelector  OutputSignals=CAN4_ZR_APM_WinRFOpened_Sta
  bus_selector38 : BusSelector  OutputSignals=CAN4_ZR_APM_WinRROpened_Sta
  bus_selector39 : BusSelector  OutputSignals=CAN4_ZR_PSEAT_Error_Sta
  bus_selector4 : BusSelector  OutputSignals=CAN3_Fr_MotorAvailTq
  bus_selector40 : BusSelector  OutputSignals=CAN4_ZR_PSEAT_Mode_Sta
  bus_selector41 : BusSelector  OutputSignals=CAN4_ZR_PSEAT_Vent_Sta
  bus_selector42 : BusSelector  OutputSignals=CAN4_ZR_PSEAT_heater_Sta
  bus_selector43 : BusSelector  OutputSignals=CAN4_ZR_PTG_Active_Sta
  bus_selector44 : BusSelector  OutputSignals=CAN4_ZR_PTG_Exist_Sta
  bus_selector45 : BusSelector  OutputSignals=CAN4_ZR_PTG_IsSetHeight_Sta
  bus_selector46 : BusSelector  OutputSignals=CAN4_ZR_PTG_Sys_Sta
  bus_selector47 : BusSelector  OutputSignals=CAN4_ZR_SEAT_LVent_Sta
  bus_selector48 : BusSelector  OutputSignals=CAN4_ZR_SEAT_MLVent_Sta
  bus_selector49 : BusSelector  OutputSignals=CAN4_ZR_SEAT_MRVent_Sta
  bus_selector5 : BusSelector  OutputSignals=CAN3_Fr_TMSpd
  bus_selector50 : BusSelector  OutputSignals=CAN4_ZR_SEAT_RVent_Sta
  bus_selector6 : BusSelector  OutputSignals=CAN3_Fr_TMTemp
  bus_selector7 : BusSelector  OutputSignals=CAN3_Fr_TMTempWarn
  bus_selector8 : BusSelector  OutputSignals=CAN3_MCU_B_F_LLCTempWarn_Sta
  bus_selector9 : BusSelector  OutputSignals=CAN3_MCU_B_R_LLCTempWarn_Sta
  P_CAN2_GW2_CE100_1 : Outport
  wires:
  bus_creator/1 -> P_CAN2_GW2_CE100_1/1
  bus_selector/1 -> bus_creator/1  "<CAN3_Fr_EDUDrtSta>"
  [R_CAN3_MCU_B_F1] -> bus_selector/1
  bus_selector1/1 -> bus_creator/2  "<CAN3_Fr_EDURealTMTq>"
  [R_CAN3_MCU_B_F1] -> bus_selector1/1
  bus_selector2/1 -> bus_creator/3  "<CAN3_Fr_MCUTemp>"
  [R_CAN3_MCU_B_F1] -> bus_selector2/1
  bus_selector3/1 -> bus_creator/4  "<CAN3_Fr_MCUTempWarn>"
  [R_CAN3_MCU_B_F2] -> bus_selector3/1
  bus_selector4/1 -> bus_creator/5  "<CAN3_Fr_MotorAvailTq>"
  [R_CAN3_MCU_B_F1] -> bus_selector4/1
  bus_selector5/1 -> bus_creator/6  "<CAN3_Fr_TMSpd>"
  [R_CAN3_MCU_B_F1] -> bus_selector5/1
  bus_selector6/1 -> bus_creator/7  "<CAN3_Fr_TMTemp>"
  [R_CAN3_MCU_B_F1] -> bus_selector6/1
  bus_selector7/1 -> bus_creator/8  "<CAN3_Fr_TMTempWarn>"
  [R_CAN3_MCU_B_F2] -> bus_selector7/1
  bus_selector8/1 -> bus_creator/9  "<CAN3_MCU_B_F_LLCTempWarn_Sta>"
  [R_CAN3_MCU_B_F2] -> bus_selector8/1
  bus_selector9/1 -> bus_creator/10  "<CAN3_MCU_B_R_LLCTempWarn_Sta>"
  [R_CAN3_MCU_B_R2] -> bus_selector9/1
  bus_selector10/1 -> bus_creator/11  "<CAN3_Rr_EDUDrtSta>"
  [R_CAN3_MCU_B_R1] -> bus_selector10/1
  bus_selector11/1 -> bus_creator/12  "<CAN3_Rr_EDURealTMTq>"
  [R_CAN3_MCU_B_R1] -> bus_selector11/1
  bus_selector12/1 -> bus_creator/13  "<CAN3_Rr_MCUTemp>"
  [R_CAN3_MCU_B_R1] -> bus_selector12/1
  bus_selector13/1 -> bus_creator/14  "<CAN3_Rr_MCUTempWarn>"
  [R_CAN3_MCU_B_R2] -> bus_selector13/1
  bus_selector14/1 -> bus_creator/15  "<CAN3_Rr_MotorAvailTq>"
  [R_CAN3_MCU_B_R1] -> bus_selector14/1
  bus_selector15/1 -> bus_creator/16  "<CAN3_Rr_TMSpd>"
  [R_CAN3_MCU_B_R1] -> bus_selector15/1
  bus_selector16/1 -> bus_creator/17  "<CAN3_Rr_TMTemp>"
  [R_CAN3_MCU_B_R1] -> bus_selector16/1
  bus_selector17/1 -> bus_creator/18  "<CAN3_Rr_TMTempWarn>"
  [R_CAN3_MCU_B_R2] -> bus_selector17/1
  bus_selector18/1 -> bus_creator/19  "<CAN4_SWC2_L_DriveMode_Sta>"
  [R_CAN4_zGW_LINDr1] -> bus_selector18/1
  bus_selector19/1 -> bus_creator/20  "<CAN4_SWC2_L_Home_Sta>"
  [R_CAN4_zGW_LINDr1] -> bus_selector19/1
  bus_selector20/1 -> bus_creator/21  "<CAN4_SWC2_R_Customize_Sta>"
  [R_CAN4_zGW_LINDr1] -> bus_selector20/1
  bus_selector21/1 -> bus_creator/22  "<CAN4_SWC2_R_Left_Sta>"
  [R_CAN4_zGW_LINDr1] -> bus_selector21/1
  bus_selector22/1 -> bus_creator/23  "<CAN4_SWC2_R_PageSwitch_Sta>"
  [R_CAN4_zGW_LINDr1] -> bus_selector22/1
  bus_selector23/1 -> bus_creator/24  "<CAN4_SWC2_R_Right_Sta>"
  [R_CAN4_zGW_LINDr1] -> bus_selector23/1
  bus_selector24/1 -> bus_creator/25  "<CAN4_SWC2_R_ScrollDown_Sta>"
  [R_CAN4_zGW_LINDr1] -> bus_selector24/1
  bus_selector25/1 -> bus_creator/26  "<CAN4_SWC2_R_ScrollPress_Sta>"
  [R_CAN4_zGW_LINDr1] -> bus_selector25/1
  bus_selector26/1 -> bus_creator/27  "<CAN4_SWC2_R_ScrollUp_Sta>"
  [R_CAN4_zGW_LINDr1] -> bus_selector26/1
  bus_selector27/1 -> bus_creator/28  "<CAN4_SWC2_R_VR_Sta>"
  [R_CAN4_zGW_LINDr1] -> bus_selector27/1
  bus_selector28/1 -> bus_creator/29  "<CAN4_ZL_APM_WinLFOpened_Sta>"
  [R_CAN4_ZONE_L2] -> bus_selector28/1
  bus_selector29/1 -> bus_creator/30  "<CAN4_ZL_APM_WinLROpened_Sta>"
  [R_CAN4_ZONE_L2] -> bus_selector29/1
  bus_selector30/1 -> bus_creator/31  "<CAN4_ZL_DSEAT_Anti_Sta>"
  [R_CAN4_ZONE_L1] -> bus_selector30/1
  bus_selector31/1 -> bus_creator/32  "<CAN4_ZL_DSEAT_EntryFun_Sta>"
  [R_CAN4_ZONE_L1] -> bus_selector31/1
  bus_selector32/1 -> bus_creator/33  "<CAN4_ZL_DSEAT_Error_Sta>"
  [R_CAN4_ZONE_L1] -> bus_selector32/1
  bus_selector33/1 -> bus_creator/34  "<CAN4_ZL_DSEAT_MemSet_Sta>"
  [R_CAN4_ZONE_L1] -> bus_selector33/1
  bus_selector34/1 -> bus_creator/35  "<CAN4_ZL_DSEAT_Mode_Sta>"
  [R_CAN4_ZONE_L1] -> bus_selector34/1
  bus_selector35/1 -> bus_creator/36  "<CAN4_ZL_DSEAT_Vent_Sta>"
  [R_CAN4_ZONE_L1] -> bus_selector35/1
  bus_selector36/1 -> bus_creator/37  "<CAN4_ZL_DSEAT_heater_Sta>"
  [R_CAN4_ZONE_L1] -> bus_selector36/1
  bus_selector37/1 -> bus_creator/38  "<CAN4_ZR_APM_WinRFOpened_Sta>"
  [R_CAN4_ZONE_R2] -> bus_selector37/1
  bus_selector38/1 -> bus_creator/39  "<CAN4_ZR_APM_WinRROpened_Sta>"
  [R_CAN4_ZONE_R2] -> bus_selector38/1
  bus_selector39/1 -> bus_creator/40  "<CAN4_ZR_PSEAT_Error_Sta>"
  [R_CAN4_ZONE_R1] -> bus_selector39/1
  bus_selector40/1 -> bus_creator/41  "<CAN4_ZR_PSEAT_Mode_Sta>"
  [R_CAN4_ZONE_R1] -> bus_selector40/1
  bus_selector41/1 -> bus_creator/42  "<CAN4_ZR_PSEAT_Vent_Sta>"
  [R_CAN4_ZONE_R1] -> bus_selector41/1
  bus_selector42/1 -> bus_creator/43  "<CAN4_ZR_PSEAT_heater_Sta>"
  [R_CAN4_ZONE_R1] -> bus_selector42/1
  bus_selector43/1 -> bus_creator/44  "<CAN4_ZR_PTG_Active_Sta>"
  [R_CAN4_ZONE_R1] -> bus_selector43/1
  bus_selector44/1 -> bus_creator/45  "<CAN4_ZR_PTG_Exist_Sta>"
  [R_CAN4_ZONE_R1] -> bus_selector44/1
  bus_selector45/1 -> bus_creator/46  "<CAN4_ZR_PTG_IsSetHeight_Sta>"
  [R_CAN4_ZONE_R1] -> bus_selector45/1
  bus_selector46/1 -> bus_creator/47  "<CAN4_ZR_PTG_Sys_Sta>"
  [R_CAN4_ZONE_R1] -> bus_selector46/1
  bus_selector47/1 -> bus_creator/48  "<CAN4_ZR_SEAT_LVent_Sta>"
  [R_CAN4_ZONE_R2] -> bus_selector47/1
  bus_selector48/1 -> bus_creator/49  "<CAN4_ZR_SEAT_MLVent_Sta>"
  [R_CAN4_ZONE_R2] -> bus_selector48/1
  bus_selector49/1 -> bus_creator/50  "<CAN4_ZR_SEAT_MRVent_Sta>"
  [R_CAN4_ZONE_R2] -> bus_selector49/1
  bus_selector50/1 -> bus_creator/51  "<CAN4_ZR_SEAT_RVent_Sta>"
  [R_CAN4_ZONE_R2] -> bus_selector50/1
  R_CAN3_MCU_B_F1/1 -> [R_CAN3_MCU_B_F1]
  R_CAN3_MCU_B_F2/1 -> [R_CAN3_MCU_B_F2]
  R_CAN3_MCU_B_R1/1 -> [R_CAN3_MCU_B_R1]
  R_CAN3_MCU_B_R2/1 -> [R_CAN3_MCU_B_R2]
  R_CAN4_ZONE_L1/1 -> [R_CAN4_ZONE_L1]
  R_CAN4_ZONE_L2/1 -> [R_CAN4_ZONE_L2]
  R_CAN4_ZONE_R1/1 -> [R_CAN4_ZONE_R1]
  R_CAN4_ZONE_R2/1 -> [R_CAN4_ZONE_R2]
  R_CAN4_zGW_LINDr1/1 -> [R_CAN4_zGW_LINDr1]

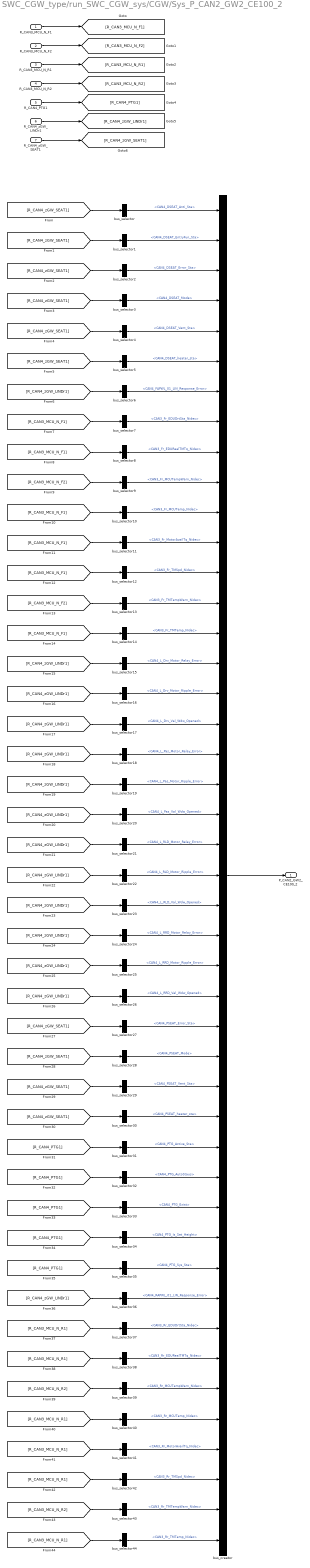
== system SWC_CGW_type/run_SWC_CGW_sys/CGW/Sys_P_CAN2_GW2_CE100_2 ==
  R_CAN3_MCU_N_F1 : Inport
  R_CAN3_MCU_N_F2 : Inport  Port=2
  R_CAN3_MCU_N_R1 : Inport  Port=3
  R_CAN3_MCU_N_R2 : Inport  Port=4
  R_CAN4_PTG1 : Inport  Port=5
  R_CAN4_zGW_LINDr1 : Inport  Port=6
  R_CAN4_zGW_SEAT1 : Inport  Port=7
  bus_creator : BusCreator  Inputs=45  OutDataTypeStr=Bus: DT_CAN2_SG_GW2_CE100_2  NonVirtualBus=on
  bus_selector : BusSelector  OutputSignals=CAN4_DSEAT_Anti_Sta
  bus_selector1 : BusSelector  OutputSignals=CAN4_DSEAT_EntryFun_Sta
  bus_selector10 : BusSelector  OutputSignals=CAN3_Fr_MCUTemp_Nidec
  bus_selector11 : BusSelector  OutputSignals=CAN3_Fr_MotorAvailTq_Nidec
  bus_selector12 : BusSelector  OutputSignals=CAN3_Fr_TMSpd_Nidec
  bus_selector13 : BusSelector  OutputSignals=CAN3_Fr_TMTempWarn_Nidec
  bus_selector14 : BusSelector  OutputSignals=CAN3_Fr_TMTemp_Nidec
  bus_selector15 : BusSelector  OutputSignals=CAN4_L_Drv_Motor_Relay_Error
  bus_selector16 : BusSelector  OutputSignals=CAN4_L_Drv_Motor_Ripple_Error
  bus_selector17 : BusSelector  OutputSignals=CAN4_L_Drv_Val_Wdw_Opened
  bus_selector18 : BusSelector  OutputSignals=CAN4_L_Pas_Motor_Relay_Error
  bus_selector19 : BusSelector  OutputSignals=CAN4_L_Pas_Motor_Ripple_Error
  bus_selector2 : BusSelector  OutputSignals=CAN4_DSEAT_Error_Sta
  bus_selector20 : BusSelector  OutputSignals=CAN4_L_Pas_Val_Wdw_Opened
  bus_selector21 : BusSelector  OutputSignals=CAN4_L_RLD_Motor_Relay_Error
  bus_selector22 : BusSelector  OutputSignals=CAN4_L_RLD_Motor_Ripple_Error
  bus_selector23 : BusSelector  OutputSignals=CAN4_L_RLD_Val_Wdw_Opened
  bus_selector24 : BusSelector  OutputSignals=CAN4_L_RRD_Motor_Relay_Error
  bus_selector25 : BusSelector  OutputSignals=CAN4_L_RRD_Motor_Ripple_Error
  bus_selector26 : BusSelector  OutputSignals=CAN4_L_RRD_Val_Wdw_Opened
  bus_selector27 : BusSelector  OutputSignals=CAN4_PSEAT_Error_Sta
  bus_selector28 : BusSelector  OutputSignals=CAN4_PSEAT_Mode
  bus_selector29 : BusSelector  OutputSignals=CAN4_PSEAT_Vent_Sta
  bus_selector3 : BusSelector  OutputSignals=CAN4_DSEAT_Mode
  bus_selector30 : BusSelector  OutputSignals=CAN4_PSEAT_heater_sta
  bus_selector31 : BusSelector  OutputSignals=CAN4_PTG_Active_Sta
  bus_selector32 : BusSelector  OutputSignals=CAN4_PTG_AutoStaus
  bus_selector33 : BusSelector  OutputSignals=CAN4_PTG_Exist
  bus_selector34 : BusSelector  OutputSignals=CAN4_PTG_Is_Set_Height
  bus_selector35 : BusSelector  OutputSignals=CAN4_PTG_Sys_Sta
  bus_selector36 : BusSelector  OutputSignals=CAN4_RAPWL_01_LIN_Response_Error
  bus_selector37 : BusSelector  OutputSignals=CAN3_Rr_EDUDrtSta_Nidec
  bus_selector38 : BusSelector  OutputSignals=CAN3_Rr_EDURealTMTq_Nidec
  bus_selector39 : BusSelector  OutputSignals=CAN3_Rr_MCUTempWarn_Nidec
  bus_selector4 : BusSelector  OutputSignals=CAN4_DSEAT_Vent_Sta
  bus_selector40 : BusSelector  OutputSignals=CAN3_Rr_MCUTemp_Nidec
  bus_selector41 : BusSelector  OutputSignals=CAN3_Rr_MotorAvailTq_Nidec
  bus_selector42 : BusSelector  OutputSignals=CAN3_Rr_TMSpd_Nidec
  bus_selector43 : BusSelector  OutputSignals=CAN3_Rr_TMTempWarn_Nidec
  bus_selector44 : BusSelector  OutputSignals=CAN3_Rr_TMTemp_Nidec
  bus_selector5 : BusSelector  OutputSignals=CAN4_DSEAT_heater_sta
  bus_selector6 : BusSelector  OutputSignals=CAN4_FAPWL_01_LIN_Response_Error
  bus_selector7 : BusSelector  OutputSignals=CAN3_Fr_EDUDrtSta_Nidec
  bus_selector8 : BusSelector  OutputSignals=CAN3_Fr_EDURealTMTq_Nidec
  bus_selector9 : BusSelector  OutputSignals=CAN3_Fr_MCUTempWarn_Nidec
  P_CAN2_GW2_CE100_2 : Outport
  wires:
  bus_creator/1 -> P_CAN2_GW2_CE100_2/1
  bus_selector/1 -> bus_creator/1  "<CAN4_DSEAT_Anti_Sta>"
  [R_CAN4_zGW_SEAT1] -> bus_selector/1
  bus_selector1/1 -> bus_creator/2  "<CAN4_DSEAT_EntryFun_Sta>"
  [R_CAN4_zGW_SEAT1] -> bus_selector1/1
  bus_selector2/1 -> bus_creator/3  "<CAN4_DSEAT_Error_Sta>"
  [R_CAN4_zGW_SEAT1] -> bus_selector2/1
  bus_selector3/1 -> bus_creator/4  "<CAN4_DSEAT_Mode>"
  [R_CAN4_zGW_SEAT1] -> bus_selector3/1
  bus_selector4/1 -> bus_creator/5  "<CAN4_DSEAT_Vent_Sta>"
  [R_CAN4_zGW_SEAT1] -> bus_selector4/1
  bus_selector5/1 -> bus_creator/6  "<CAN4_DSEAT_heater_sta>"
  [R_CAN4_zGW_SEAT1] -> bus_selector5/1
  bus_selector6/1 -> bus_creator/7  "<CAN4_FAPWL_01_LIN_Response_Error>"
  [R_CAN4_zGW_LINDr1] -> bus_selector6/1
  bus_selector7/1 -> bus_creator/8  "<CAN3_Fr_EDUDrtSta_Nidec>"
  [R_CAN3_MCU_N_F1] -> bus_selector7/1
  bus_selector8/1 -> bus_creator/9  "<CAN3_Fr_EDURealTMTq_Nidec>"
  [R_CAN3_MCU_N_F1] -> bus_selector8/1
  bus_selector9/1 -> bus_creator/10  "<CAN3_Fr_MCUTempWarn_Nidec>"
  [R_CAN3_MCU_N_F2] -> bus_selector9/1
  bus_selector10/1 -> bus_creator/11  "<CAN3_Fr_MCUTemp_Nidec>"
  [R_CAN3_MCU_N_F1] -> bus_selector10/1
  bus_selector11/1 -> bus_creator/12  "<CAN3_Fr_MotorAvailTq_Nidec>"
  [R_CAN3_MCU_N_F1] -> bus_selector11/1
  bus_selector12/1 -> bus_creator/13  "<CAN3_Fr_TMSpd_Nidec>"
  [R_CAN3_MCU_N_F1] -> bus_selector12/1
  bus_selector13/1 -> bus_creator/14  "<CAN3_Fr_TMTempWarn_Nidec>"
  [R_CAN3_MCU_N_F2] -> bus_selector13/1
  bus_selector14/1 -> bus_creator/15  "<CAN3_Fr_TMTemp_Nidec>"
  [R_CAN3_MCU_N_F1] -> bus_selector14/1
  bus_selector15/1 -> bus_creator/16  "<CAN4_L_Drv_Motor_Relay_Error>"
  [R_CAN4_zGW_LINDr1] -> bus_selector15/1
  bus_selector16/1 -> bus_creator/17  "<CAN4_L_Drv_Motor_Ripple_Error>"
  [R_CAN4_zGW_LINDr1] -> bus_selector16/1
  bus_selector17/1 -> bus_creator/18  "<CAN4_L_Drv_Val_Wdw_Opened>"
  [R_CAN4_zGW_LINDr1] -> bus_selector17/1
  bus_selector18/1 -> bus_creator/19  "<CAN4_L_Pas_Motor_Relay_Error>"
  [R_CAN4_zGW_LINDr1] -> bus_selector18/1
  bus_selector19/1 -> bus_creator/20  "<CAN4_L_Pas_Motor_Ripple_Error>"
  [R_CAN4_zGW_LINDr1] -> bus_selector19/1
  bus_selector20/1 -> bus_creator/21  "<CAN4_L_Pas_Val_Wdw_Opened>"
  [R_CAN4_zGW_LINDr1] -> bus_selector20/1
  bus_selector21/1 -> bus_creator/22  "<CAN4_L_RLD_Motor_Relay_Error>"
  [R_CAN4_zGW_LINDr1] -> bus_selector21/1
  bus_selector22/1 -> bus_creator/23  "<CAN4_L_RLD_Motor_Ripple_Error>"
  [R_CAN4_zGW_LINDr1] -> bus_selector22/1
  bus_selector23/1 -> bus_creator/24  "<CAN4_L_RLD_Val_Wdw_Opened>"
  [R_CAN4_zGW_LINDr1] -> bus_selector23/1
  bus_selector24/1 -> bus_creator/25  "<CAN4_L_RRD_Motor_Relay_Error>"
  [R_CAN4_zGW_LINDr1] -> bus_selector24/1
  bus_selector25/1 -> bus_creator/26  "<CAN4_L_RRD_Motor_Ripple_Error>"
  [R_CAN4_zGW_LINDr1] -> bus_selector25/1
  bus_selector26/1 -> bus_creator/27  "<CAN4_L_RRD_Val_Wdw_Opened>"
  [R_CAN4_zGW_LINDr1] -> bus_selector26/1
  bus_selector27/1 -> bus_creator/28  "<CAN4_PSEAT_Error_Sta>"
  [R_CAN4_zGW_SEAT1] -> bus_selector27/1
  bus_selector28/1 -> bus_creator/29  "<CAN4_PSEAT_Mode>"
  [R_CAN4_zGW_SEAT1] -> bus_selector28/1
  bus_selector29/1 -> bus_creator/30  "<CAN4_PSEAT_Vent_Sta>"
  [R_CAN4_zGW_SEAT1] -> bus_selector29/1
  bus_selector30/1 -> bus_creator/31  "<CAN4_PSEAT_heater_sta>"
  [R_CAN4_zGW_SEAT1] -> bus_selector30/1
  bus_selector31/1 -> bus_creator/32  "<CAN4_PTG_Active_Sta>"
  [R_CAN4_PTG1] -> bus_selector31/1
  bus_selector32/1 -> bus_creator/33  "<CAN4_PTG_AutoStaus>"
  [R_CAN4_PTG1] -> bus_selector32/1
  bus_selector33/1 -> bus_creator/34  "<CAN4_PTG_Exist>"
  [R_CAN4_PTG1] -> bus_selector33/1
  bus_selector34/1 -> bus_creator/35  "<CAN4_PTG_Is_Set_Height>"
  [R_CAN4_PTG1] -> bus_selector34/1
  bus_selector35/1 -> bus_creator/36  "<CAN4_PTG_Sys_Sta>"
  [R_CAN4_PTG1] -> bus_selector35/1
  bus_selector36/1 -> bus_creator/37  "<CAN4_RAPWL_01_LIN_Response_Error>"
  [R_CAN4_zGW_LINDr1] -> bus_selector36/1
  bus_selector37/1 -> bus_creator/38  "<CAN3_Rr_EDUDrtSta_Nidec>"
  [R_CAN3_MCU_N_R1] -> bus_selector37/1
  bus_selector38/1 -> bus_creator/39  "<CAN3_Rr_EDURealTMTq_Nidec>"
  [R_CAN3_MCU_N_R1] -> bus_selector38/1
  bus_selector39/1 -> bus_creator/40  "<CAN3_Rr_MCUTempWarn_Nidec>"
  [R_CAN3_MCU_N_R2] -> bus_selector39/1
  bus_selector40/1 -> bus_creator/41  "<CAN3_Rr_MCUTemp_Nidec>"
  [R_CAN3_MCU_N_R1] -> bus_selector40/1
  bus_selector41/1 -> bus_creator/42  "<CAN3_Rr_MotorAvailTq_Nidec>"
  [R_CAN3_MCU_N_R1] -> bus_selector41/1
  bus_selector42/1 -> bus_creator/43  "<CAN3_Rr_TMSpd_Nidec>"
  [R_CAN3_MCU_N_R1] -> bus_selector42/1
  bus_selector43/1 -> bus_creator/44  "<CAN3_Rr_TMTempWarn_Nidec>"
  [R_CAN3_MCU_N_R2] -> bus_selector43/1
  bus_selector44/1 -> bus_creator/45  "<CAN3_Rr_TMTemp_Nidec>"
  [R_CAN3_MCU_N_R1] -> bus_selector44/1
  R_CAN3_MCU_N_F1/1 -> [R_CAN3_MCU_N_F1]
  R_CAN3_MCU_N_F2/1 -> [R_CAN3_MCU_N_F2]
  R_CAN3_MCU_N_R1/1 -> [R_CAN3_MCU_N_R1]
  R_CAN3_MCU_N_R2/1 -> [R_CAN3_MCU_N_R2]
  R_CAN4_PTG1/1 -> [R_CAN4_PTG1]
  R_CAN4_zGW_LINDr1/1 -> [R_CAN4_zGW_LINDr1]
  R_CAN4_zGW_SEAT1/1 -> [R_CAN4_zGW_SEAT1]
